simulink library "NMEA"  (R2024a)
settings: Solver=VariableStepAuto  StartTime=0.0  StopTime=10.0  RelTol=1e-3
libraries: $bdroot x44, simulink x21, simulink_extras x17, etargetslib x14
(part 4 of 4)

== matlab function NMEA/Details/NMEA Checksum Message/MATLAB Function ==
  data: nmeaData input; bytes output; len output
function [bytes, len] = CreateMessage(nmeaData)
    BUFFER_SIZE = uint32(128);

    % Default output values
    bytes = uint8(zeros(BUFFER_SIZE,1));
    len = uint32(0);

    % Compute checksum
    data = uint8(char(nmeaData))';
    datalen = length(data);
    cs = uint8(0);
    for i = 2:(datalen-1)
        cs = bitxor(cs, data(i));
    end
    msb = bitand(bitshift(cs,-4),uint8(15));
    lsb = bitand(cs,uint8(15));
    if(msb < 10), msb = msb + uint8(48); else, msb = msb + uint8(55); end
    if(lsb < 10), lsb = lsb + uint8(48); else, lsb = lsb + uint8(55); end

    % Add checksum
    if(uint32(datalen + 2) <= BUFFER_SIZE)
        bytes(1:datalen) = data;
        bytes(datalen + 1) = msb;
        bytes(datalen + 2) = lsb;
        len = uint32(datalen + 2);
    end
end
